simulink model "power_PSS"  (Simulink 6.0)
settings: Solver=ode23tb  StartTime=0.0  StopTime=20  MaxStep=1/60  RelTol=1e-4
undefined symbols (not defined in the file or in its folder): D1, Delta
libraries: powerlib x49, powerlib_extras x4
settings Model: Creator=rchampag  LastModifiedBy=batserve  ExtModeTrigMode=oneshot  ExtModeArmWhenConnect=off  ExtModeAutoUpdateStatusClock=off
settings DataIOCC: LimitDataPoints=off  SaveOutput=off  SaveTime=off  TimeSaveName=t  SignalLoggingName=sigsOut
settings OptimizationCC: BlockReduction=off  BooleanDataType=off
settings DebuggingCC: SolverPrmCheckMsg=none  UnconnectedOutputMsg=none
settings HardwareCC: TargetUnknown=on

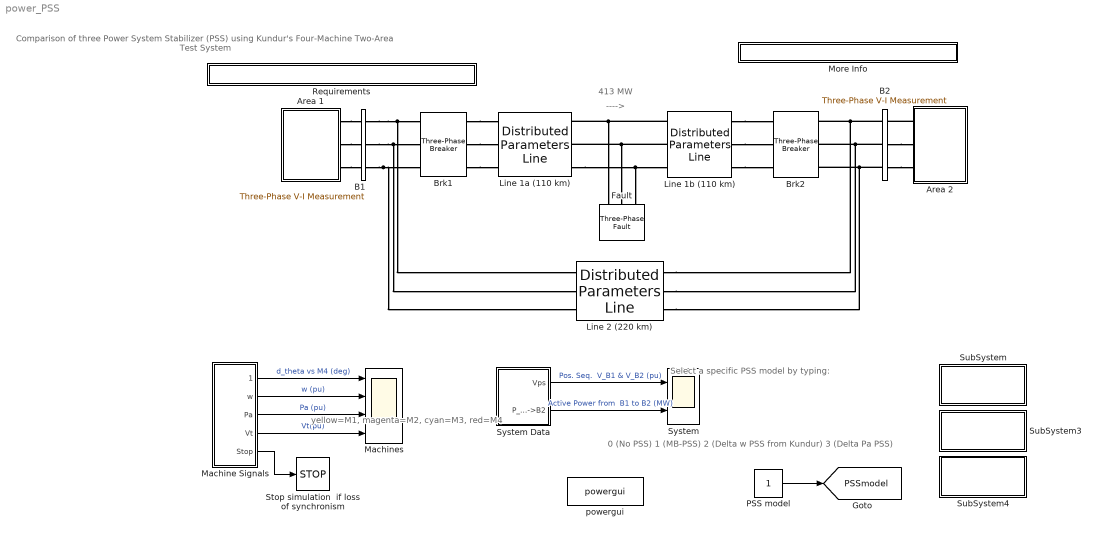
== system power_PSS ==
  note: Comparison of three Power System Stabilizer (PSS)
      | using Kundur's Four-Machine Two-Area Test System
  note: yellow=M1,
      | magenta=M2,
      | cyan=M3,
      | red=M4
  note: ---->
  note: 413 MW
  note: Select a specific PSS model
      | by typing:
  note: 0  (No PSS)
      | 1  (MB-PSS)
      | 2  (Delta w PSS from Kundur)
      | 3  (Delta Pa PSS)
  " Brk2" : powerlib/Elements/Three-Phase Breaker  InitialState=closed  SwitchA=on  SwitchB=on  SwitchC=on  SwitchTimes=[1+8/60]  External=off  BreakerResistance=0.001  SnubberResistance=1e6  SnubberCapacitance=0  Measurements=None
      settings: AttributesFormatString=\n
  Area 1 : Subsystem
  Area 2 : Subsystem
  B1 : powerlib/Measurements/Three-Phase V-I Measurement  VoltageMeasurement=phase-to-ground  SetLabelV=on  LabelV=Vabc_B1  Vpu=off  Vbase=500e3  CurrentMeasurement=yes  SetLabelI=on  LabelI=Iabc_B1  Ipu=off  Pbase=100e6  OutputType=Complex  PhasorSimulation=on  PSBequivalent=0
  B2 : powerlib/Measurements/Three-Phase V-I Measurement  VoltageMeasurement=phase-to-ground  SetLabelV=on  LabelV=Vabc_B2  Vpu=off  Vbase=500e3  CurrentMeasurement=yes  SetLabelI=on  LabelI=Iabc_B2  Ipu=off  Pbase=100e6  OutputType=Complex  PhasorSimulation=on  PSBequivalent=0
  Brk1 : powerlib/Elements/Three-Phase Breaker  InitialState=closed  SwitchA=on  SwitchB=on  SwitchC=on  SwitchTimes=[1+8/60]  External=off  BreakerResistance=0.001  SnubberResistance=inf  SnubberCapacitance=0  Measurements=None
      settings: AttributesFormatString=\n
  Fault : powerlib/Elements/Three-Phase Fault  Orientation=down  FaultA=on  FaultB=on  FaultC=on  FaultResistance=0.001  GroundFault=on  GroundResistance=0.001  External=off  SwitchStatus=[1 0]  SwitchTimes=[ 1 1+12/60]  InitialStates=[0 0 1]  SnubberResistance=inf  SnubberCapacitance=0  Measurements=None
  Line 1a (110 km) : powerlib/Elements/Distributed Parameters Line  Phases=3  Frequency=60  Resistance=[0.0001*529 1.61]  Inductance=[0.001*529/(377) 0.0061]  Capacitance=[0.00175/529/(377) 5.2489e-9]  Length=110  x1=[0 -1.08e-008 1.364e+005 -1.828e+005;0.0001245 -1.04e-008 1.448e+005 -1.762e+005;0.000249 -9.969e-009 1.529e+005 -1.692e+005;0.0003735 -9.519e-009 1.607e+005 -1.618e+005;0.0004979 -9.048e-009 1.681e+005 -1.541e+005;0.0006224 -8.557e-009 1.751e+005 -1.461e+005]  x2=[0 -8.707e-009 8.941e+004 -2.072e+005;0.0001245 -8.096e-009 9.903e+004 -2.027e+005;0.000249 -7.467e-009 1.084e+005 -1.979e+005;0.0003735 -6.821e-009 1.176e+005 -1.926e+005;0.0004979 -6.16e-009 1.265e+005 -1.868e+005;0.0006224 -5.486e-009 1.351e+005 -1.807e+005]  x3=[0 -1.712e-011 -188.2 278.4;0.0001245 -1.624e-011 -201 269.2;0.000249 -1.531e-011 -213.4 259.5;0.0003735 -1.435e-011 -225.4 249.2;0.0004979 -1.336e-011 -236.8 238.4;0.0006224 -1.234e-011 -247.8 227]  x4=[0 -1.348e-012 676.1 -1284;0.0001245 -1.525e-012 735.6 -1251;0.000249 -1.7e-012 793.5 -1215;0.0003735 -1.87e-012 849.6 -1176;0.0004979 -2.037e-012 903.8 -1135;0.0006224 -2.199e-012 956.1 -1091]  x5=0.0006224  Measurements=None
      settings: AttributesFormatString=\n
  Line 1b (110 km) : powerlib/Elements/Distributed Parameters Line  Phases=3  Frequency=60  Resistance=[0.0001*529 1.61]  Inductance=[0.001*529/(377) 0.0061]  Capacitance=[0.00175/529/(377) 5.2489e-9]  Length=110  x1=[0 -8.707e-009 8.941e+004 -2.072e+005;0.0001245 -8.096e-009 9.903e+004 -2.027e+005;0.000249 -7.467e-009 1.084e+005 -1.979e+005;0.0003735 -6.821e-009 1.176e+005 -1.926e+005;0.0004979 -6.16e-009 1.265e+005 -1.868e+005;0.0006224 -5.486e-009 1.351e+005 -1.807e+005]  x2=[0 -6.602e-009 4.098e+004 -2.27e+005;0.0001245 -5.796e-009 5.158e+004 -2.248e+005;0.000249 -4.976e-009 6.207e+004 -2.221e+005;0.0003735 -4.146e-009 7.242e+004 -2.19e+005;0.0004979 -3.306e-009 8.262e+004 -2.153e+005;0.0006224 -2.459e-009 9.263e+004 -2.112e+005]  x3=[0 -1.532e-011 -233.8 258.9;0.0001245 -1.425e-011 -245.7 247.7;0.000249 -1.315e-011 -257 235.9;0.0003735 -1.203e-011 -267.8 223.6;0.0004979 -1.088e-011 -278 210.7;0.0006224 -9.699e-012 -287.6 197.5]  x4=[0 -3.575e-013 477.8 -1356;0.0001245 -3.081e-013 540.9 -1332;0.000249 -2.58e-013 602.8 -1306;0.0003735 -2.073e-013 663.4 -1276;0.0004979 -1.562e-013 722.5 -1243;0.0006224 -1.047e-013 780 -1208]  x5=0.0006224  Measurements=None
      settings: AttributesFormatString=\n
  Line 2 (220 km) : powerlib/Elements/Distributed Parameters Line  Phases=3  Frequency=60  Resistance=[0.0001*529 1.61]  Inductance=[0.001*529/(377) 0.0061]  Capacitance=[0.00175/529/(377) 5.2489e-9]  Length=220  x1=[0 -1.135e-008 1.084e+005 -2.006e+005;0.000249 -1.036e-008 1.268e+005 -1.896e+005;0.0004979 -9.29e-009 1.44e+005 -1.769e+005;0.0007469 -8.134e-009 1.599e+005 -1.626e+005;0.0009959 -6.906e-009 1.745e+005 -1.469e+005;0.001245 -5.617e-009 1.875e+005 -1.299e+005]  x2=[0 -8.979e-009 7634 -2.305e+005;0.000249 -7.841e-009 2.92e+004 -2.288e+005;0.0004979 -6.634e-009 5.052e+004 -2.25e+005;0.0007469 -5.368e-009 7.139e+004 -2.193e+005;0.0009959 -4.055e-009 9.163e+004 -2.117e+005;0.001245 -2.707e-009 1.111e+005 -2.021e+005]  x3=[0 -1.027e-011 -145.5 302.4;0.000249 -9.359e-012 -173.2 287.5;0.0004979 -8.367e-012 -199.4 270;0.0007469 -7.303e-012 -223.8 250.1;0.0009959 -6.174e-012 -246.3 228;0.001245 -4.99e-012 -266.6 203.9]  x4=[0 -8.487e-012 273.7 -1399;0.000249 -8.24e-012 403.7 -1367;0.0004979 -7.92e-012 530 -1323;0.0007469 -7.531e-012 651.7 -1268;0.0009959 -7.075e-012 767.7 -1201;0.001245 -6.557e-012 876.9 -1124]  x5=0.001245  Measurements=None
      settings: AttributesFormatString=\n
  Machine Signals : Subsystem
  Machines : Scope  NumInputPorts=4
      settings: TimeRange=10  YMin=0~0.994~-0.35~0.95  YMax=130~1.005~0.2~1.175  SaveName=mach
  More Info : Subsystem
      settings: OpenFcn=web(which('psbpss.html'))
      mask Display: disp('? : Double click here for more info')
  PSS model : Constant
  Requirements : Subsystem  Description=|  LoadFcn=|  InitFcn=|
      LoadFcn=|
      | Toolboxes = ver;                                                                                                                 
      | installedtoolboxes = {Toolboxes.Name};                                                                                           
      | k = strcmp('Control System Toolbox',installedtoolboxes);                                                                         
      | if ~any(k)                                                                                                                       
      |     H = warndlg(['You need to install the Control System Toolbox in order to run the power_pss demo'],'SimPowerSystems warning');
      |     uiwait(H);                                                                                                                   
      | end
      InitFcn=|
      | Toolboxes = ver;                                                                                  
      | installedtoolboxes = {Toolboxes.Name};                                                            
      | k = strcmp('Control System Toolbox',installedtoolboxes);                                          
      | if ~any(k)                                                                                        
      |     error(['You need to install the Control System Toolbox in order to run the power_pss demo.']);
      | end
      Description=|
      | This block is used to popup errors and warnings if the
      | Control System Toolbox is not installed.
      settings: OpenFcn=|
      | Toolboxes = ver;
      | installedtoolboxes = {Toolboxes.Name};
      | k = strcmp('Control System Toolbox',installedtoolboxes);
      | if ~any(k)
      |     warndlg(['You need to install the Control System Toolbox in order to run the power_pss demo.'],'SimPowerSystems warning');
      |                                                                                                                                                         end
      mask Display: disp('This demo requires the Control System Toolbox')
  Stop simulation  if loss of synchronism : Stop
  SubSystem : Subsystem
      settings: OpenFcn=openfig('psbPSSbode.fig');
      mask Display: disp('Show Bode plot \nof PSS')
  SubSystem3 : Subsystem
      settings: OpenFcn=openfig('psbPSSstep.fig');
      mask Display: disp('Show results: \nStep on vref\nof M1')
  SubSystem4 : Subsystem
      settings: OpenFcn=openfig('psbPSSfault.fig');
      mask Display: disp('Show results: \n3-phase fault')
  System : Scope  NumInputPorts=2
      settings: TimeRange=10  YMin=0.9475~389  YMax=0.9675~401  SaveName=mach1
  System Data : Subsystem
  powergui : powerlib/powergui  Priority=2  Frange=logspace(0,3,50)  Ylog=off  Xlog=off  save=off  variable=ZData  ZoomFFT=on  StartTime=0.0  cycles=1  DisplayStyle=1  fundamental=60  FreqAxis=off  MaxFrequency=1000  frequencyindice=1  frequencyindicesteady=1  RmsSteady=1  display=off  Ts=0  methode=on  frequency=60  echomessages=on
  tag scope: PSSmodel=global
  wires:
  Machine Signals/1(d_theta) -> Machines/1  "d_theta vs M4 (deg)"
  Machine Signals/2(w) -> Machines/2  "w (pu)"
  Machine Signals/3(Pa) -> Machines/3  "Pa (pu)"
  Machine Signals/4(Vt) -> Machines/4  "Vt(pu)"
  Machine Signals/5(Stop) -> Stop simulation  if loss of synchronism/1
  System Data/1(Vps) -> System/1  "Pos. Seq.  V_B1 & V_B2 (pu)"
  System Data/2(P_B1->B2) -> System/2  "Active Power from  B1 to B2 (MW)"
  PSS model/1 -> [PSSmodel]
  connections:
  Brk1/RConn1 -- Line 1a (110 km)/LConn1
  Brk1/RConn2 -- Line 1a (110 km)/LConn2
  Brk1/RConn3 -- Line 1a (110 km)/LConn3
  Line 1b (110 km)/LConn1 -- Line 1a (110 km)/RConn1 -- Fault/LConn1
  Line 1b (110 km)/LConn2 -- Line 1a (110 km)/RConn2 -- Fault/LConn2
  Line 1a (110 km)/RConn3 -- Line 1b (110 km)/LConn3 -- Fault/LConn3
  Line 1b (110 km)/RConn1 -- " Brk2"/LConn1
  Line 1b (110 km)/RConn2 -- " Brk2"/LConn2
  Line 1b (110 km)/RConn3 -- " Brk2"/LConn3
  Area 1/RConn2 -- B1/LConn2
  Area 1/RConn1 -- B1/LConn1
  Area 1/RConn3 -- B1/LConn3
  B1/RConn2 -- Brk1/LConn2 -- Line 2 (220 km)/LConn2
  B1/RConn1 -- Brk1/LConn1 -- Line 2 (220 km)/LConn1
  B1/RConn3 -- Brk1/LConn3 -- Line 2 (220 km)/LConn3
  B2/RConn2 -- Area 2/LConn2
  Area 2/LConn1 -- B2/RConn1
  B2/RConn3 -- Area 2/LConn3
  B2/LConn2 -- " Brk2"/RConn2 -- Line 2 (220 km)/RConn2
  B2/LConn1 -- " Brk2"/RConn1 -- Line 2 (220 km)/RConn1
  B2/LConn3 -- " Brk2"/RConn3 -- Line 2 (220 km)/RConn3

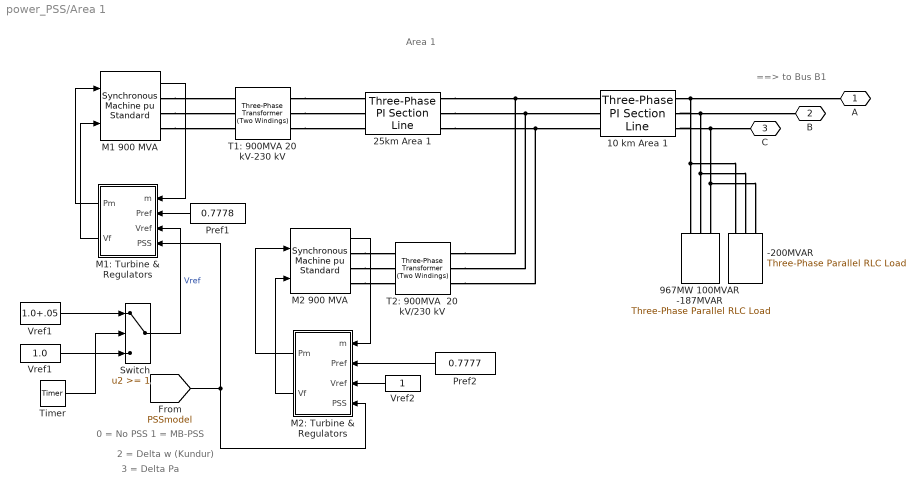
== system power_PSS/Area 1 ==
  note: Area 1
  note: ==> to Bus B1
  note: 0 = No PSS
      | 1 = MB-PSS
  note: 3 = Delta Pa
  note: 2 = Delta w (Kundur)
  -200MVAR : powerlib/Elements/Three-Phase Parallel RLC Load  Orientation=down  PhysicalDomain=powersysdomain  SubClassName=unknown  LeftPortType=p1  RightPortType=p1  LConnTagsString=A|B|C  Configuration=Y (grounded)  NominalVoltage=230e3  NominalFrequency=60  ActivePower=0  InductivePower=0  CapacitivePower=200e6  Measurements=None
  10 km Area 1 : powerlib/Elements/Three-Phase PI Section Line  PhysicalDomain=powersysdomain  SubClassName=unknown  LeftPortType=p1  RightPortType=p1  LConnTagsString=a|b|c  RConnTagsString=A|B|C  Frequency=60  Resistances=[0.0001*529 1.61]  Inductances=[0.001*529/(377) 0.0061]  Capacitances=[0.00175/529/(377) 5.2489e-9]  Length=10
  25km Area 1 : powerlib/Elements/Three-Phase PI Section Line  PhysicalDomain=powersysdomain  SubClassName=unknown  LeftPortType=p1  RightPortType=p1  LConnTagsString=a|b|c  RConnTagsString=A|B|C  Frequency=60  Resistances=[0.0001*529 1.61]  Inductances=[0.001*529/(377) 0.0061]  Capacitances=[0.00175/529/(377) 5.2489e-9]  Length=25
  967MW 100MVAR -187MVAR : powerlib/Elements/Three-Phase Parallel RLC Load  Orientation=down  PhysicalDomain=powersysdomain  SubClassName=unknown  LeftPortType=p1  RightPortType=p1  LConnTagsString=A|B|C  Configuration=Y (grounded)  NominalVoltage=230e3  NominalFrequency=60  ActivePower=967e6  InductivePower=100e6  CapacitivePower=187e6  Measurements=None
  M1 900 MVA : powerlib/Machines/Synchronous Machine pu Standard  PresetModel=No  ShowDetailedParameters=on  RotorType=Round  NominalParameters="[900E6  20000   60 ]"  Reactances1=[1.8 .3 .25 1.7 .55 .25 .2]  Reactances2=[ 1.305, 0.296, 0.252, 0.474, 0.243, 0.18 ]  dAxisTimeConstants=Open-circuit  qAxisTimeConstants=Open-circuit  TimeConstants1=[]  TimeConstants2=[8 .03 .4 .05]  TimeConstants3=[]  TimeConstants4=[]  TimeConstants5=[ 1.01, 0.053, 0.1 ]  TimeConstants6=[]  TimeConstants7=[]  TimeConstants8=[]  StatorResistance=0.0025  Mechanical="[ 6.5 0  4]"  InitialConditions=[0 -31.4247 0.784453 0.784453 0.784453 2.7401 -117.26 122.74 1.83395]  SetSaturation=off  Saturation=[0.6404,0.7127,0.8441,0.9214,0.9956,1.082,1.19,1.316,1.457;0.7,0.7698,0.8872,0.9466,0.9969,1.046,1.1,1.151,1.201]  Units=0.5  LoadFlowParameters=[1 700000000 0 0 0]
      settings: AttributesFormatString=\n\n
  M1: Turbine & Regulators : Subsystem  Orientation=left
  M2 900 MVA : powerlib/Machines/Synchronous Machine pu Standard  PresetModel=No  ShowDetailedParameters=on  RotorType=Round  NominalParameters="[900E6  20000   60 ]"  Reactances1=[1.8 .3 .25 1.7 .55 .25 .2]  Reactances2=[ 1.305, 0.296, 0.252, 0.474, 0.243, 0.18 ]  dAxisTimeConstants=Open-circuit  qAxisTimeConstants=Open-circuit  TimeConstants1=[]  TimeConstants2=[8 .03 .4 .05]  TimeConstants3=[]  TimeConstants4=[]  TimeConstants5=[ 1.01, 0.053, 0.1 ]  TimeConstants6=[]  TimeConstants7=[]  TimeConstants8=[]  StatorResistance=0.0025  Mechanical="[ 6.5 0  4]"  InitialConditions=[0 -42.8075 0.788608 0.788608 0.788608 -9.54571 -129.546 110.454 1.86756]  SetSaturation=off  Saturation=[0.6404,0.7127,0.8441,0.9214,0.9956,1.082,1.19,1.316,1.457;0.7,0.7698,0.8872,0.9466,0.9969,1.046,1.1,1.151,1.201]  Units=0.5  LoadFlowParameters=[2 700000000 0 0 0]
      settings: AttributesFormatString=\n\n
  M2: Turbine & Regulators : Subsystem  Orientation=left
  Pref1 : Constant  Orientation=left  Value=0.7778
  Pref2 : Constant  Orientation=left  Value=0.7777
  Switch : Switch  Threshold=1  InputSameDT=on
  T1: 900MVA 20 kV-230 kV : powerlib/Elements/Three-Phase Transformer (Two Windings)  NominalPower="[ 900e6   60 ]"  Winding1Connection=Delta (D1)  Winding1="[ 20e3  1e-6   0  ]"  Winding2Connection=Yg  Winding2="[ 230e3  1e-6   0.15 ]"  SetSaturation=off  Rm=500  Lm=500  Saturation="[ 0,0  ;  0.005,1.2  ;  1.0,1.4 ]"  Hysteresis=off  DataFile='hysteresis'  SetInitialFlux=off  InitialFluxes=[ 0.8 , -0.8 , 0.7 ]  Measurements=None  TransfoNumber=0
  T2: 900MVA  20 kV/230 kV : powerlib/Elements/Three-Phase Transformer (Two Windings)  NominalPower=[ 900e6 60 ]  Winding1Connection=Delta (D1)  Winding1="[ 20e3 1e-6  0.0]"  Winding2Connection=Yg  Winding2=[ 230e3 1e-6 0.15]  SetSaturation=off  Rm=500  Lm=500  Saturation="[ 0,0  ;  0.005,1.2  ;  1.0,1.4 ]"  Hysteresis=off  DataFile='hysteresis'  SetInitialFlux=off  InitialFluxes=[ 0.8 , -0.8 , 0.7 ]  Measurements=None  TransfoNumber=0
  Timer : powerlib_extras/Control  Blocks/Timer  t=[0 1 1.2]*100  e=[0 1 0 ]
  Vref1 : Constant  Value=1.0
  "Vref1 " : Constant  Value=1.0+.05
  Vref2 : Constant  Orientation=left
  " A" : PMIOPort  Orientation=left  Port=1  Side=Right
  " B" : PMIOPort  Orientation=left  Port=2  Side=Right
  " C" : PMIOPort  Orientation=left  Port=3  Side=Right
  wires:
  Pref1/1 -> M1: Turbine & Regulators/2(Pref)
  Switch/1 -> M1: Turbine & Regulators/3(Vref)  "Vref"
  Timer/1 -> Switch/2
  [PSSmodel] -> M1: Turbine & Regulators/4(PSS), M2: Turbine & Regulators/4(PSS)
  Pref2/1 -> M2: Turbine & Regulators/2(Pref)
  Vref2/1 -> M2: Turbine & Regulators/3(Vref)
  Vref1/1 -> Switch/3
  "Vref1 "/1 -> Switch/1
  M2 900 MVA/1 -> M2: Turbine & Regulators/1(m)
  M2: Turbine & Regulators/1(Pm) -> M2 900 MVA/1
  M2: Turbine & Regulators/2(Vf) -> M2 900 MVA/2
  M1: Turbine & Regulators/1(Pm) -> M1 900 MVA/1
  M1: Turbine & Regulators/2(Vf) -> M1 900 MVA/2
  M1 900 MVA/1 -> M1: Turbine & Regulators/1(m)
  connections:
  T1: 900MVA 20 kV-230 kV/RConn1 -- 25km Area 1/LConn1
  T1: 900MVA 20 kV-230 kV/RConn2 -- 25km Area 1/LConn2
  M2 900 MVA/RConn1 -- T2: 900MVA  20 kV/230 kV/LConn1
  M2 900 MVA/RConn2 -- T2: 900MVA  20 kV/230 kV/LConn2
  M2 900 MVA/RConn3 -- T2: 900MVA  20 kV/230 kV/LConn3
  T1: 900MVA 20 kV-230 kV/RConn3 -- 25km Area 1/LConn3
  10 km Area 1/RConn1 -- " A"/RConn1 -- 967MW 100MVAR -187MVAR/LConn1 -- -200MVAR/LConn1
  10 km Area 1/RConn2 -- " B"/RConn1 -- 967MW 100MVAR -187MVAR/LConn2 -- -200MVAR/LConn2
  10 km Area 1/RConn3 -- " C"/RConn1 -- 967MW 100MVAR -187MVAR/LConn3 -- -200MVAR/LConn3
  M1 900 MVA/RConn1 -- T1: 900MVA 20 kV-230 kV/LConn1
  M1 900 MVA/RConn2 -- T1: 900MVA 20 kV-230 kV/LConn2
  M1 900 MVA/RConn3 -- T1: 900MVA 20 kV-230 kV/LConn3
  25km Area 1/RConn2 -- 10 km Area 1/LConn2 -- T2: 900MVA  20 kV/230 kV/RConn2
  25km Area 1/RConn1 -- 10 km Area 1/LConn1 -- T2: 900MVA  20 kV/230 kV/RConn1
  25km Area 1/RConn3 -- 10 km Area 1/LConn3 -- T2: 900MVA  20 kV/230 kV/RConn3

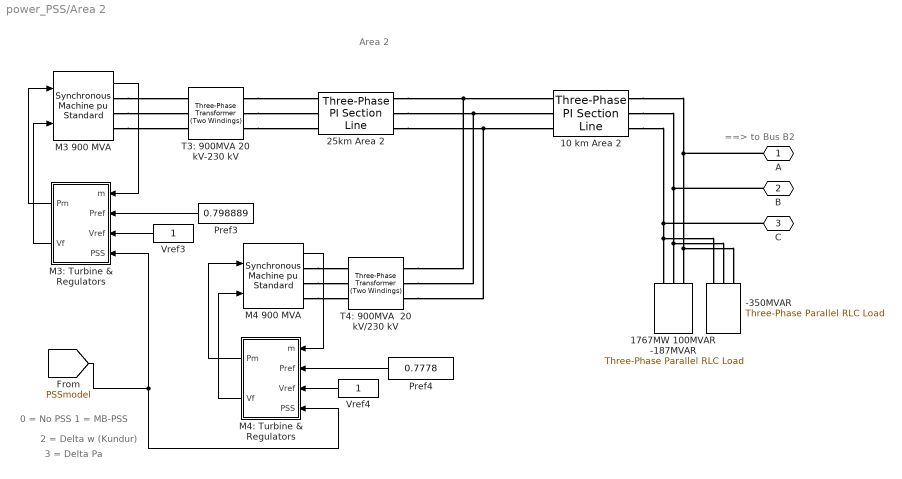
== system power_PSS/Area 2 ==
  note: 2 = Delta w (Kundur)
  note: 3 = Delta Pa
  note: 0 = No PSS
      | 1 = MB-PSS
  note: ==> to Bus B2
  note: Area 2
  -350MVAR : powerlib/Elements/Three-Phase Parallel RLC Load  Orientation=down  PhysicalDomain=powersysdomain  SubClassName=unknown  LeftPortType=p1  RightPortType=p1  LConnTagsString=A|B|C  Configuration=Y (grounded)  NominalVoltage=230e3  NominalFrequency=60  ActivePower=0  InductivePower=0  CapacitivePower=350e6  Measurements=None
  10 km Area 2 : powerlib/Elements/Three-Phase PI Section Line  PhysicalDomain=powersysdomain  SubClassName=unknown  LeftPortType=p1  RightPortType=p1  LConnTagsString=a|b|c  RConnTagsString=A|B|C  Frequency=60  Resistances=[0.0001*529 1.61]  Inductances=[0.001*529/(377) 0.0061]  Capacitances=[0.00175/529/(377) 5.2489e-9]  Length=10
  1767MW 100MVAR -187MVAR : powerlib/Elements/Three-Phase Parallel RLC Load  Orientation=down  PhysicalDomain=powersysdomain  SubClassName=unknown  LeftPortType=p1  RightPortType=p1  LConnTagsString=A|B|C  Configuration=Y (grounded)  NominalVoltage=230e3  NominalFrequency=60  ActivePower=1767e6  InductivePower=100e6  CapacitivePower=187e6  Measurements=None
  25km Area 2 : powerlib/Elements/Three-Phase PI Section Line  PhysicalDomain=powersysdomain  SubClassName=unknown  LeftPortType=p1  RightPortType=p1  LConnTagsString=a|b|c  RConnTagsString=A|B|C  Frequency=60  Resistances=[0.0001*529 1.61]  Inductances=[0.001*529/(377) 0.0061]  Capacitances=[0.00175/529/(377) 5.2489e-9]  Length=25
  M3 900 MVA : powerlib/Machines/Synchronous Machine pu Standard  PresetModel=No  ShowDetailedParameters=on  RotorType=Round  NominalParameters="[900E6  20000   60 ]"  Reactances1=[1.8 .3 .25 1.7 .55 .25 .2]  Reactances2=[ 1.305, 0.296, 0.252, 0.474, 0.243, 0.18 ]  dAxisTimeConstants=Open-circuit  qAxisTimeConstants=Open-circuit  TimeConstants1=[]  TimeConstants2=[8 .03 .4 .05]  TimeConstants3=[]  TimeConstants4=[]  TimeConstants5=[ 1.01, 0.053, 0.1 ]  TimeConstants6=[]  TimeConstants7=[]  TimeConstants8=[]  StatorResistance=0.0025  Mechanical="[ 6.175 0  4]"  InitialConditions=[0 -56.3243 0.8041 0.8041 0.8041 -22.4087 -142.409 97.5913 1.85092]  SetSaturation=off  Saturation=[0.6404,0.7127,0.8441,0.9214,0.9956,1.082,1.19,1.316,1.457;0.7,0.7698,0.8872,0.9466,0.9969,1.046,1.1,1.151,1.201]  Units=0.5  LoadFlowParameters=[1 719000000 0 0 0]
      settings: AttributesFormatString=\n\n
  M3: Turbine & Regulators : Subsystem  Orientation=left
  M4 900 MVA : powerlib/Machines/Synchronous Machine pu Standard  PresetModel=No  ShowDetailedParameters=on  RotorType=Round  NominalParameters="[900E6  20000   60 ]"  Reactances1=[1.8 .3 .25 1.7 .55 .25 .2]  Reactances2=[ 1.305, 0.296, 0.252, 0.474, 0.243, 0.18 ]  dAxisTimeConstants=Open-circuit  qAxisTimeConstants=Open-circuit  TimeConstants1=[]  TimeConstants2=[8 .03 .4 .05]  TimeConstants3=[]  TimeConstants4=[]  TimeConstants5=[ 1.01, 0.053, 0.1 ]  TimeConstants6=[]  TimeConstants7=[]  TimeConstants8=[]  StatorResistance=0.0025  Mechanical="[ 6.175 0  4]"  InitialConditions=[0 -67.7513 0.783185 0.783185 0.783185 -33.268 -153.268 86.732 1.82209]  SetSaturation=off  Saturation=[0.6404,0.7127,0.8441,0.9214,0.9956,1.082,1.19,1.316,1.457;0.7,0.7698,0.8872,0.9466,0.9969,1.046,1.1,1.151,1.201]  Units=0.5  LoadFlowParameters=[1 700000000 0 0 0]
      settings: AttributesFormatString=\n\n
  M4: Turbine & Regulators : Subsystem  Orientation=left
  Pref3 : Constant  Orientation=left  Value=0.798889
  Pref4 : Constant  Orientation=left  Value=0.7778
  T3: 900MVA 20 kV-230 kV : powerlib/Elements/Three-Phase Transformer (Two Windings)  NominalPower="[ 900e6   60 ]"  Winding1Connection=Delta (D1)  Winding1="[ 20e3  1e-6   0  ]"  Winding2Connection=Yg  Winding2="[ 230e3  1e-6   0.15 ]"  SetSaturation=off  Rm=500  Lm=500  Saturation="[ 0,0  ;  0.005,1.2  ;  1.0,1.4 ]"  Hysteresis=off  DataFile='hysteresis'  SetInitialFlux=off  InitialFluxes=[ 0.8 , -0.8 , 0.7 ]  Measurements=None  TransfoNumber=0
  T4: 900MVA  20 kV/230 kV : powerlib/Elements/Three-Phase Transformer (Two Windings)  NominalPower=[ 900e6 60 ]  Winding1Connection=Delta (D1)  Winding1="[ 20e3 1e-6  0.0]"  Winding2Connection=Yg  Winding2=[ 230e3 1e-6 0.15]  SetSaturation=off  Rm=500  Lm=500  Saturation="[ 0,0  ;  0.005,1.2  ;  1.0,1.4 ]"  Hysteresis=off  DataFile='hysteresis'  SetInitialFlux=off  InitialFluxes=[ 0.8 , -0.8 , 0.7 ]  Measurements=None  TransfoNumber=0
  Vref3 : Constant  Orientation=left
  Vref4 : Constant  Orientation=left
  A : PMIOPort  Orientation=left  Port=1  Side=Left
  B : PMIOPort  Orientation=left  Port=2  Side=Left
  C : PMIOPort  Orientation=left  Port=3  Side=Left
  wires:
  [PSSmodel] -> M3: Turbine & Regulators/4(PSS), M4: Turbine & Regulators/4(PSS)
  Pref3/1 -> M3: Turbine & Regulators/2(Pref)
  Vref3/1 -> M3: Turbine & Regulators/3(Vref)
  Pref4/1 -> M4: Turbine & Regulators/2(Pref)
  Vref4/1 -> M4: Turbine & Regulators/3(Vref)
  M3 900 MVA/1 -> M3: Turbine & Regulators/1(m)
  M3: Turbine & Regulators/2(Vf) -> M3 900 MVA/2
  M3: Turbine & Regulators/1(Pm) -> M3 900 MVA/1
  M4: Turbine & Regulators/1(Pm) -> M4 900 MVA/1
  M4: Turbine & Regulators/2(Vf) -> M4 900 MVA/2
  M4 900 MVA/1 -> M4: Turbine & Regulators/1(m)
  connections:
  M3 900 MVA/RConn3 -- T3: 900MVA 20 kV-230 kV/LConn3
  M3 900 MVA/RConn2 -- T3: 900MVA 20 kV-230 kV/LConn2
  M3 900 MVA/RConn1 -- T3: 900MVA 20 kV-230 kV/LConn1
  T3: 900MVA 20 kV-230 kV/RConn3 -- 25km Area 2/LConn3
  M4 900 MVA/RConn3 -- T4: 900MVA  20 kV/230 kV/LConn3
  M4 900 MVA/RConn2 -- T4: 900MVA  20 kV/230 kV/LConn2
  M4 900 MVA/RConn1 -- T4: 900MVA  20 kV/230 kV/LConn1
  T3: 900MVA 20 kV-230 kV/RConn2 -- 25km Area 2/LConn2
  T3: 900MVA 20 kV-230 kV/RConn1 -- 25km Area 2/LConn1
  10 km Area 2/RConn1 -- A/RConn1 -- 1767MW 100MVAR -187MVAR/LConn3 -- -350MVAR/LConn3
  10 km Area 2/RConn2 -- B/RConn1 -- 1767MW 100MVAR -187MVAR/LConn2 -- -350MVAR/LConn2
  10 km Area 2/RConn3 -- C/RConn1 -- 1767MW 100MVAR -187MVAR/LConn1 -- -350MVAR/LConn1
  25km Area 2/RConn2 -- 10 km Area 2/LConn2 -- T4: 900MVA  20 kV/230 kV/RConn2
  25km Area 2/RConn1 -- 10 km Area 2/LConn1 -- T4: 900MVA  20 kV/230 kV/RConn1
  25km Area 2/RConn3 -- 10 km Area 2/LConn3 -- T4: 900MVA  20 kV/230 kV/RConn3

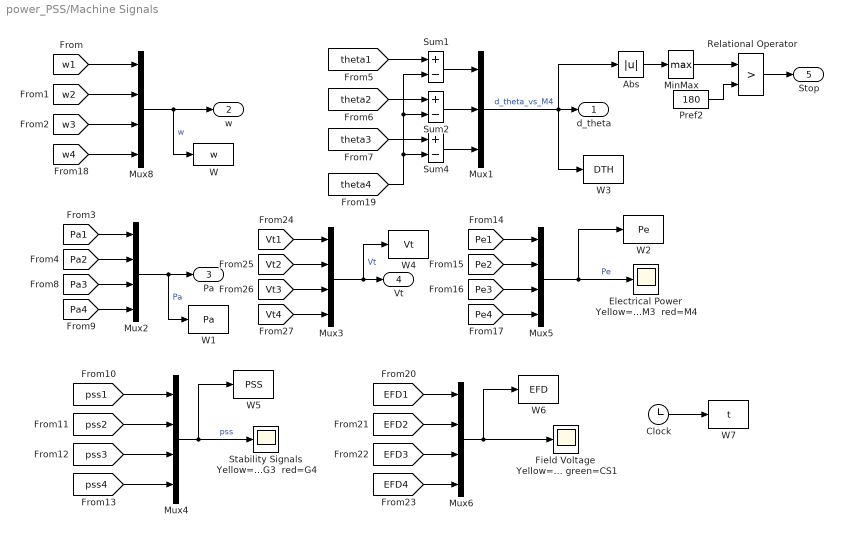
== system power_PSS/Machine Signals ==
  Abs : Abs  SaturateOnIntegerOverflow=on
  Clock : Clock
      settings: Decimation=10
  "Electrical Power  Yellow=M1 mag=M2 cyan=M3  red=M4 " : Scope
      settings: YMin=0.3  YMax=1
  Field Voltage  Yellow=G1 mag=G2 cyan=G3  red=G4 green=CS1 : Scope
      settings: YMin=1.845  YMax=1.96  SaveName=ScopeData4
  MinMax : MinMax  Function=max  SaturateOnIntegerOverflow=on  InputSameDT=on
  Mux1 : Mux  Inputs=3
  Mux{2..6,8} (6 alike) : Mux
  Pref2 : Constant  Value=180
  Relational Operator : RelationalOperator  Operator=>  InputSameDT=on
  "Stability Signals  Yellow=G1 mag=G2 cyan=G3  red=G4 " : Scope
      settings: YMin=-0.15  YMax=0.15  SaveName=ScopeData3
  Sum1 : Sum  Inputs=+-  SaturateOnIntegerOverflow=on  InputSameDT=on
  Sum2 : Sum  Inputs=+-  SaturateOnIntegerOverflow=on  InputSameDT=on
  Sum4 : Sum  Inputs=+-  SaturateOnIntegerOverflow=on  InputSameDT=on
  W : ToWorkspace  VariableName=w  SampleTime=1/60  SaveFormat=Array
  W1 : ToWorkspace  VariableName=Pa  SampleTime=1/60  SaveFormat=Array
  W2 : ToWorkspace  VariableName=Pe  SampleTime=1/60  SaveFormat=Array
  W3 : ToWorkspace  VariableName=DTH  SampleTime=1/60  SaveFormat=Array
  W4 : ToWorkspace  VariableName=Vt  SampleTime=1/60  SaveFormat=Array
  W5 : ToWorkspace  VariableName=PSS  SampleTime=1/60  SaveFormat=Array
  W6 : ToWorkspace  VariableName=EFD  SampleTime=1/60  SaveFormat=Array
  W7 : ToWorkspace  VariableName=t  SampleTime=1/60  SaveFormat=Array
  d_theta : Outport
  w : Outport  Port=2
  Pa : Outport  Port=3
  Vt : Outport  Port=4
  Stop : Outport  Port=5
  wires:
  Mux1/1 -> d_theta/1, Abs/1, W3/1  "d_theta_vs_M4"
  Abs/1 -> MinMax/1
  Pref2/1 -> Relational Operator/2
  MinMax/1 -> Relational Operator/1
  [Pa1] -> Mux2/1
  Mux4/1 -> "Stability Signals  Yellow=G1 mag=G2 cyan=G3  red=G4 "/1, W5/1  "pss"
  [pss1] -> Mux4/1
  [pss2] -> Mux4/2
  [pss4] -> Mux4/4
  [pss3] -> Mux4/3
  [EFD1] -> Mux6/1
  [EFD2] -> Mux6/2
  [EFD4] -> Mux6/4
  [EFD3] -> Mux6/3
  Mux6/1 -> Field Voltage  Yellow=G1 mag=G2 cyan=G3  red=G4 green=CS1/1, W6/1
  Mux8/1 -> w/1, W/1  "w"
  Relational Operator/1 -> Stop/1
  Mux2/1 -> Pa/1, W1/1  "Pa"
  [theta1] -> Sum1/1
  Sum1/1 -> Mux1/1
  [theta2] -> Sum2/1
  [theta3] -> Sum4/1
  [theta4] -> Sum4/2, Sum2/2, Sum1/2
  Sum2/1 -> Mux1/2
  Sum4/1 -> Mux1/3
  [Pa2] -> Mux2/2
  [Pa3] -> Mux2/3
  [Pa4] -> Mux2/4
  [Vt1] -> Mux3/1
  [Vt2] -> Mux3/2
  [Vt3] -> Mux3/3
  [Vt4] -> Mux3/4
  Mux3/1 -> Vt/1, W4/1  "Vt"
  [Pe1] -> Mux5/1
  [Pe2] -> Mux5/2
  [Pe3] -> Mux5/3
  [Pe4] -> Mux5/4
  Mux5/1 -> "Electrical Power  Yellow=M1 mag=M2 cyan=M3  red=M4 "/1, W2/1  "Pe"
  [w1] -> Mux8/1
  [w2] -> Mux8/2
  [w3] -> Mux8/3
  [w4] -> Mux8/4
  Clock/1 -> W7/1

== system power_PSS/More Info ==

== system power_PSS/Requirements ==

== system power_PSS/SubSystem ==

== system power_PSS/SubSystem3 ==

== system power_PSS/SubSystem4 ==

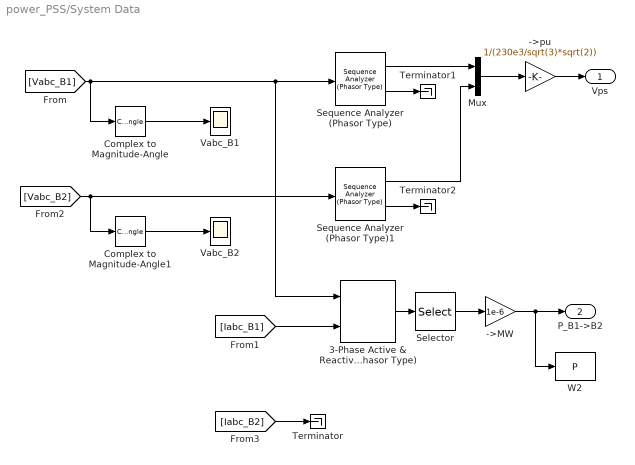
== system power_PSS/System Data ==
  ->MW : Gain  Gain=1e-6  SaturateOnIntegerOverflow=on
  ->pu : Gain  Gain=1/(230e3/sqrt(3)*sqrt(2))  SaturateOnIntegerOverflow=on
  3-Phase Active & Reactive Power (Phasor Type) : powerlib_extras/Phasor Library/3-Phase Active & Reactive Power (Phasor Type)
  Complex to Magnitude-Angle : ComplexToMagnitudeAngle  Output=Magnitude
  Complex to Magnitude-Angle1 : ComplexToMagnitudeAngle  Output=Magnitude
  Mux : Mux  Inputs=2
  Selector : Selector  InputPortWidth=2
  Sequence Analyzer (Phasor Type) : powerlib_extras/Phasor Library/Sequence Analyzer (Phasor Type)  seq=Positive
  Sequence Analyzer (Phasor Type)1 : powerlib_extras/Phasor Library/Sequence Analyzer (Phasor Type)  seq=Positive
  Terminator : Terminator
  Terminator1 : Terminator
  Terminator2 : Terminator
  Vabc_B1 : Scope
      settings: TimeRange=10  YMin=20  YMax=90  SaveName=mach2
  Vabc_B2 : Scope
      settings: TimeRange=10  YMin=20  YMax=90  SaveName=mach3
  W2 : ToWorkspace  VariableName=P  SampleTime=1/60  SaveFormat=Array
  Vps : Outport
  P_B1->B2 : Outport  Port=2
  wires:
  [Vabc_B1] -> Sequence Analyzer (Phasor Type)/1, 3-Phase Active & Reactive Power (Phasor Type)/1, Complex to Magnitude-Angle/1
  [Vabc_B2] -> Sequence Analyzer (Phasor Type)1/1, Complex to Magnitude-Angle1/1
  [Iabc_B2] -> Terminator/1
  Sequence Analyzer (Phasor Type)/2 -> Terminator1/1
  Sequence Analyzer (Phasor Type)1/2 -> Terminator2/1
  Sequence Analyzer (Phasor Type)1/1 -> Mux/2
  [Iabc_B1] -> 3-Phase Active & Reactive Power (Phasor Type)/2
  3-Phase Active & Reactive Power (Phasor Type)/1 -> Selector/1
  ->pu/1 -> Vps/1
  Sequence Analyzer (Phasor Type)/1 -> Mux/1
  Mux/1 -> ->pu/1
  ->MW/1 -> P_B1->B2/1, W2/1
  Complex to Magnitude-Angle/1 -> Vabc_B1/1
  Complex to Magnitude-Angle1/1 -> Vabc_B2/1
  Selector/1 -> ->MW/1

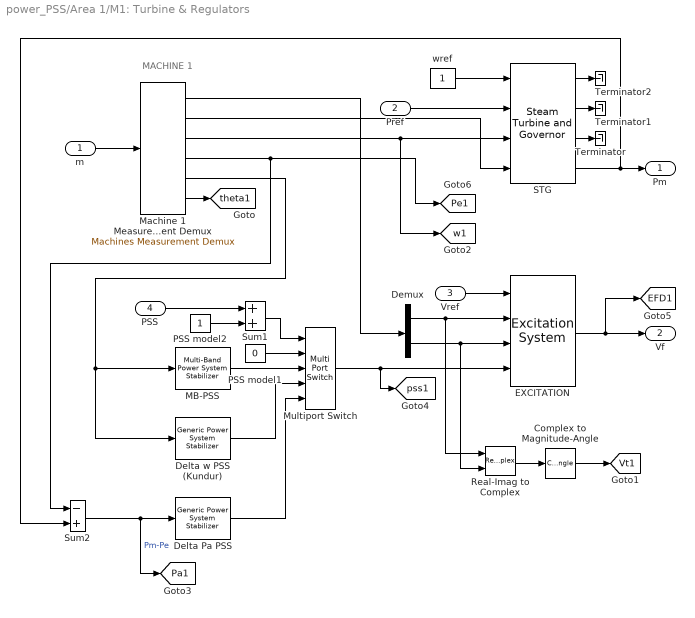
== system power_PSS/Area 1/M1: Turbine & Regulators ==
  note: MACHINE 1
  m : Inport  Port=1  LatchInput=off
  Pref : Inport  Port=2  LatchInput=off
  Vref : Inport  Port=3  LatchInput=off
  PSS : Inport  Port=4  LatchInput=off
  Complex to Magnitude-Angle : ComplexToMagnitudeAngle  Output=Magnitude
  "Delta Pa PSS " : powerlib/Machines/Generic Power System Stabilizer  Tsensor=15e-3  K=2.5*1.25  Twashout=1  Tleadlag1=[60e-3 1]  Tleadlag2=[0 0]  VSlimits=[-0.15 0.15]  Vinit=0  Plot_On=off  MagdB_On=off  FreqRange=logspace(-2,2,500)
  "Delta w PSS (Kundur) " : powerlib/Machines/Generic Power System Stabilizer  Tsensor=15e-3  K=30  Twashout=10  Tleadlag1=[50e-3 20e-3]  Tleadlag2=[3 5.4]  VSlimits=[-0.15 0.15]  Vinit=0  Plot_On=off  MagdB_On=off  FreqRange=logspace(-2,2,500)
  Demux : Demux  Outputs=2
  EXCITATION : powerlib/Machines/Excitation System  tr=20e-3  reg=[ 200, 0.001 ]  exc=[ 1, 0 ]  tgr=[ 0, 0 ]  damp=[ 0, 0 ]  sat=[ 0, 0 ]  lim=[ 0 , 12.3, 0 ]  v0=[1,1.83395]
  "MB-PSS " : powerlib/Machines/Multi-Band Power System Stabilizer  OperationMode=Simplified settings  Kg=1.0  GL=[0.2 30]  GI=[1.25 40]  GH=[12.0 160]  GLd=[66 66 9.4]  TcLF=[1.667 2 0 0 0 0 2 2.4 0 0 0 0 1 1]  GId=[66 66 47.6]  TcIF=[1 1 0.25 0.3 0 0 1 1 0.3 0.36 0 0 0 0]  GHd=[66 66 233]  TcHF="[0.01 0.012 0 0 0 0  0.012 0.0144 0 0 0 0 1 1]"  LIM=[.075 .15 .15 .15]  Plot_On=off  MagdB_On=off  FreqRange=logspace(-2,2,500)
  Machine 1 Measurement Demux : powerlib/Machines/Machines Measurement Demux  machType=Synchronous  ssm1=on  ssm2=on  ssm3=on  ssm4=on  ssm5=on  ssm6=on  sm1=off  sm2=off  sm3=off  sm4=off  sm5=off  sm6=on  sm7=on  sm8=on  sm9=on  sm10=on  sm11=on  sm115=off  sm12=off  sm13=off  sm14=off  asm1=on  asm2=on  asm3=on  asm4=on  asm5=on  asm6=on  asm7=on  asm8=on  asm9=on  asm10=on  asm11=on  pmsm1=on  pmsm2=on  pmsm3=on  pmsm4=on  pmsm5=on  pmsm6=on  lastType=2
  Multiport Switch : MultiPortSwitch  InputSameDT=on
  PSS model1 : Constant  Value=0
  PSS model2 : Constant
  Real-Imag to Complex : RealImagToComplex
  STG : powerlib/Machines/Steam Turbine and Governor  gentype=Tandem-compound (single mass)  reg1="[ 1  0.05    0 ]"  reg2="[ 0.001  0.15 ]"  reg3="[ -0.1  0.1  0  4.496 ]"  turb1="[ 0  10   3.3   0.5   ]"  turb2="[   0   0.36    0.36   0.28   ]"  HA="[ 0.046  1.430  1.465   0.192 ]"  KA="[ 90.44  53.88  64.59   62.94  ]"  DA="[ 0.0115  0.3575  0.3663   0.0137  ]"  ini1=0.7778  ini2=[0.779316,-31.4247]
  Sum1 : Sum  SaturateOnIntegerOverflow=on  InputSameDT=on
  Sum2 : Sum  Inputs=-+  SaturateOnIntegerOverflow=on  InputSameDT=on
  Terminator : Terminator
  Terminator1 : Terminator
  Terminator2 : Terminator
  wref : Constant
  Pm : Outport  InitialOutput=0
  Vf : Outport  Port=2  InitialOutput=0
  tag scope: EFD1=global, Pa1=global, Pe1=global, Vt1=global, pss1=global, theta1=global, w1=global
  wires:
  Demux/1 -> Real-Imag to Complex/1, EXCITATION/2
  Demux/2 -> Real-Imag to Complex/2, EXCITATION/3
  wref/1 -> STG/1
  Pref/1 -> STG/2
  m/1 -> Machine 1 Measurement Demux/1
  Vref/1 -> EXCITATION/1
  Real-Imag to Complex/1 -> Complex to Magnitude-Angle/1
  EXCITATION/1 -> Vf/1, [EFD1]
  Complex to Magnitude-Angle/1 -> [Vt1]
  Machine 1 Measurement Demux/6 -> [theta1]
  Multiport Switch/1 -> EXCITATION/4, [pss1]
  PSS model1/1 -> Multiport Switch/2
  "MB-PSS "/1 -> Multiport Switch/3
  "Delta w PSS (Kundur) "/1 -> Multiport Switch/4
  "Delta Pa PSS "/1 -> Multiport Switch/5
  PSS model2/1 -> Sum1/2
  Sum1/1 -> Multiport Switch/1
  PSS/1 -> Sum1/1
  Machine 1 Measurement Demux/1 -> Demux/1
  Machine 1 Measurement Demux/3 -> [w1], STG/3
  Machine 1 Measurement Demux/4 -> Sum2/1, [Pe1]
  Machine 1 Measurement Demux/5 -> "Delta w PSS (Kundur) "/1, "MB-PSS "/1
  Sum2/1 -> [Pa1], "Delta Pa PSS "/1  "Pm-Pe"
  STG/3 -> Terminator/1
  Machine 1 Measurement Demux/2 -> STG/4
  STG/4 -> Pm/1, Sum2/2
  STG/2 -> Terminator1/1
  STG/1 -> Terminator2/1

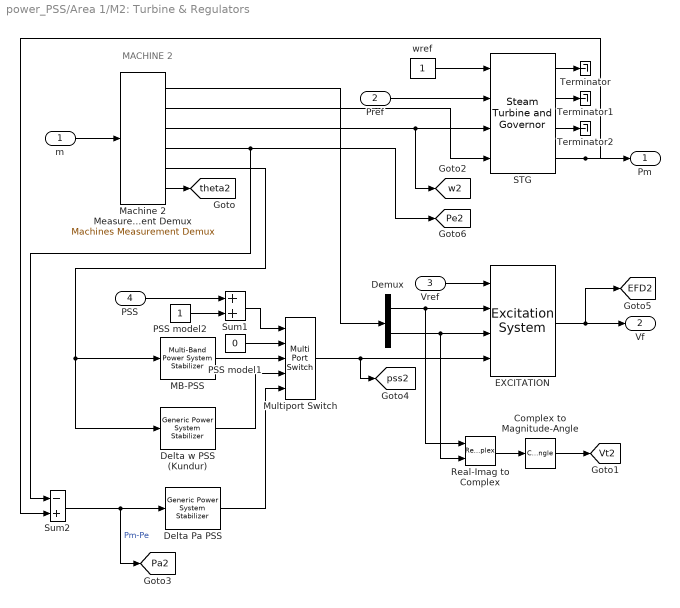
== system power_PSS/Area 1/M2: Turbine & Regulators ==
  note: MACHINE 2
  m : Inport  Port=1  LatchInput=off
  Pref : Inport  Port=2  LatchInput=off
  Vref : Inport  Port=3  LatchInput=off
  PSS : Inport  Port=4  LatchInput=off
  Complex to Magnitude-Angle : ComplexToMagnitudeAngle  Output=Magnitude
  "Delta Pa PSS " : powerlib/Machines/Generic Power System Stabilizer  Tsensor=15e-3  K=2.5*1.25  Twashout=1  Tleadlag1=[60e-3 1]  Tleadlag2=[0 0]  VSlimits=[-0.15 0.15]  Vinit=0  Plot_On=off  MagdB_On=on  FreqRange=logspace(-2,2,500)
  "Delta w PSS (Kundur) " : powerlib/Machines/Generic Power System Stabilizer  Tsensor=15e-3  K=30  Twashout=10  Tleadlag1=[50e-3 20e-3]  Tleadlag2=[3 5.4]  VSlimits=[-0.15 0.15]  Vinit=0  Plot_On=off  MagdB_On=on  FreqRange=logspace(-2,2,500)
  Demux : Demux  Outputs=2
  EXCITATION : powerlib/Machines/Excitation System  tr=20e-3  reg=[ 200, 0.001 ]  exc=[ 1, 0 ]  tgr=[ 0, 0 ]  damp=[ 0, 0 ]  sat=[ 0, 0 ]  lim=[ 0 , 12.3, 0 ]  v0=[1,1.86756]
  "MB-PSS " : powerlib/Machines/Multi-Band Power System Stabilizer  OperationMode=Simplified settings  Kg=1.0  GL=[0.2 30]  GI=[1.25 40]  GH=[12.0 160]  GLd=[66 66 9.4]  TcLF=[1.667 2 0 0 0 0 2 2.4 0 0 0 0 1 1]  GId=[66 66 47.6]  TcIF=[1 1 0.25 0.3 0 0 1 1 0.3 0.36 0 0 0 0]  GHd=[66 66 233]  TcHF="[0.01 0.012 0 0 0 0  0.012 0.0144 0 0 0 0 1 1]"  LIM=[.075 .15 .15 .15]  Plot_On=off  MagdB_On=off  FreqRange=logspace(-2,2,500)
  Machine 2 Measurement Demux : powerlib/Machines/Machines Measurement Demux  machType=Synchronous  ssm1=on  ssm2=on  ssm3=on  ssm4=on  ssm5=on  ssm6=on  sm1=off  sm2=off  sm3=off  sm4=off  sm5=off  sm6=on  sm7=on  sm8=on  sm9=on  sm10=on  sm11=on  sm115=off  sm12=off  sm13=off  sm14=off  asm1=on  asm2=on  asm3=on  asm4=on  asm5=on  asm6=on  asm7=on  asm8=on  asm9=on  asm10=on  asm11=on  pmsm1=on  pmsm2=on  pmsm3=on  pmsm4=on  pmsm5=on  pmsm6=on  lastType=2
  Multiport Switch : MultiPortSwitch  InputSameDT=on
  PSS model1 : Constant  Value=0
  PSS model2 : Constant
  Real-Imag to Complex : RealImagToComplex
  STG : powerlib/Machines/Steam Turbine and Governor  gentype=Tandem-compound (single mass)  reg1="[ 1  0.05    0 ]"  reg2="[ 0.001  0.15 ]"  reg3="[ -0.1  0.1  0  4.496 ]"  turb1="[ 0  10   3.3   0.5   ]"  turb2="[   0   0.36    0.36   0.28   ]"  HA="[ 0.046  1.430  1.465   0.192 ]"  KA="[ 90.44  53.88  64.59   62.94  ]"  DA="[ 0.0115  0.3575  0.3663   0.0137  ]"  ini1=0.7777  ini2=[0.779243,-42.8075]
  Sum1 : Sum  SaturateOnIntegerOverflow=on  InputSameDT=on
  Sum2 : Sum  Inputs=-+  SaturateOnIntegerOverflow=on  InputSameDT=on
  Terminator : Terminator
  Terminator1 : Terminator
  Terminator2 : Terminator
  wref : Constant
  Pm : Outport  InitialOutput=0
  Vf : Outport  Port=2  InitialOutput=0
  tag scope: EFD2=global, Pa2=global, Pe2=global, Vt2=global, pss2=global, theta2=global, w2=global
  wires:
  Sum2/1 -> [Pa2], "Delta Pa PSS "/1  "Pm-Pe"
  Machine 2 Measurement Demux/5 -> "MB-PSS "/1, "Delta w PSS (Kundur) "/1
  Machine 2 Measurement Demux/4 -> Sum2/1, [Pe2]
  Machine 2 Measurement Demux/3 -> [w2], STG/3
  Machine 2 Measurement Demux/1 -> Demux/1
  PSS/1 -> Sum1/1
  Sum1/1 -> Multiport Switch/1
  PSS model2/1 -> Sum1/2
  "Delta Pa PSS "/1 -> Multiport Switch/5
  "Delta w PSS (Kundur) "/1 -> Multiport Switch/4
  "MB-PSS "/1 -> Multiport Switch/3
  PSS model1/1 -> Multiport Switch/2
  Multiport Switch/1 -> [pss2], EXCITATION/4
  Machine 2 Measurement Demux/6 -> [theta2]
  Complex to Magnitude-Angle/1 -> [Vt2]
  EXCITATION/1 -> [EFD2], Vf/1
  Real-Imag to Complex/1 -> Complex to Magnitude-Angle/1
  Vref/1 -> EXCITATION/1
  m/1 -> Machine 2 Measurement Demux/1
  Pref/1 -> STG/2
  wref/1 -> STG/1
  Demux/2 -> EXCITATION/3, Real-Imag to Complex/2
  Demux/1 -> EXCITATION/2, Real-Imag to Complex/1
  STG/1 -> Terminator/1
  STG/2 -> Terminator1/1
  STG/3 -> Terminator2/1
  STG/4 -> Pm/1, Sum2/2
  Machine 2 Measurement Demux/2 -> STG/4

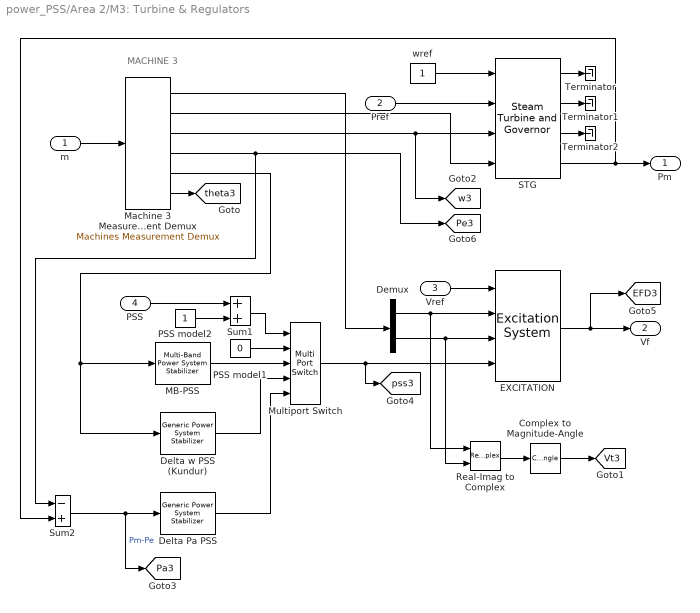
== system power_PSS/Area 2/M3: Turbine & Regulators ==
  note: MACHINE 3
  m : Inport  Port=1  LatchInput=off
  Pref : Inport  Port=2  LatchInput=off
  Vref : Inport  Port=3  LatchInput=off
  PSS : Inport  Port=4  LatchInput=off
  Complex to Magnitude-Angle : ComplexToMagnitudeAngle  Output=Magnitude
  "Delta Pa PSS " : powerlib/Machines/Generic Power System Stabilizer  Tsensor=15e-3  K=2.5*1.25  Twashout=1  Tleadlag1=[60e-3 1]  Tleadlag2=[0 0]  VSlimits=[-0.15 0.15]  Vinit=0  Plot_On=off  MagdB_On=on  FreqRange=logspace(-2,2,500)
  "Delta w PSS (Kundur) " : powerlib/Machines/Generic Power System Stabilizer  Tsensor=15e-3  K=30  Twashout=10  Tleadlag1=[50e-3 20e-3]  Tleadlag2=[3 5.4]  VSlimits=[-0.15 0.15]  Vinit=0  Plot_On=off  MagdB_On=on  FreqRange=logspace(-2,2,500)
  Demux : Demux  Outputs=2
  EXCITATION : powerlib/Machines/Excitation System  tr=20e-3  reg=[ 200, 0.001 ]  exc=[ 1, 0 ]  tgr=[ 0, 0 ]  damp=[ 0, 0 ]  sat=[ 0, 0 ]  lim=[ 0 , 12.3, 0 ]  v0=[1,1.85092]
  "MB-PSS " : powerlib/Machines/Multi-Band Power System Stabilizer  OperationMode=Simplified settings  Kg=1.0  GL=[0.2 30]  GI=[1.25 40]  GH=[12.0 160]  GLd=[66 66 9.4]  TcLF=[1.667 2 0 0 0 0 2 2.4 0 0 0 0 1 1]  GId=[66 66 47.6]  TcIF=[1 1 0.25 0.3 0 0 1 1 0.3 0.36 0 0 0 0]  GHd=[66 66 233]  TcHF="[0.01 0.012 0 0 0 0  0.012 0.0144 0 0 0 0 1 1]"  LIM=[.075 .15 .15 .15]  Plot_On=off  MagdB_On=off  FreqRange=logspace(-2,2,500)
  Machine 3 Measurement Demux : powerlib/Machines/Machines Measurement Demux  machType=Synchronous  ssm1=on  ssm2=on  ssm3=on  ssm4=on  ssm5=on  ssm6=on  sm1=off  sm2=off  sm3=off  sm4=off  sm5=off  sm6=on  sm7=on  sm8=on  sm9=on  sm10=on  sm11=on  sm115=off  sm12=off  sm13=off  sm14=off  asm1=on  asm2=on  asm3=on  asm4=on  asm5=on  asm6=on  asm7=on  asm8=on  asm9=on  asm10=on  asm11=on  pmsm1=on  pmsm2=on  pmsm3=on  pmsm4=on  pmsm5=on  pmsm6=on  lastType=2
  Multiport Switch : MultiPortSwitch  InputSameDT=on
  PSS model1 : Constant  Value=0
  PSS model2 : Constant
  Real-Imag to Complex : RealImagToComplex
  STG : powerlib/Machines/Steam Turbine and Governor  gentype=Tandem-compound (single mass)  reg1="[ 1  0.05    0 ]"  reg2="[ 0.001  0.15 ]"  reg3="[ -0.1  0.1  0  4.496 ]"  turb1="[ 0  10   3.3   0.5   ]"  turb2="[   0   0.36    0.36   0.28   ]"  HA="[ 0.046  1.430  1.465   0.192 ]"  KA="[ 90.44  53.88  64.59   62.94  ]"  DA="[ 0.0115  0.3575  0.3663   0.0137  ]"  ini1=0.798889  ini2=[0.800505,-56.3243]
  Sum1 : Sum  SaturateOnIntegerOverflow=on  InputSameDT=on
  Sum2 : Sum  Inputs=-+  SaturateOnIntegerOverflow=on  InputSameDT=on
  Terminator : Terminator
  Terminator1 : Terminator
  Terminator2 : Terminator
  wref : Constant
  Pm : Outport  InitialOutput=0
  Vf : Outport  Port=2  InitialOutput=0
  tag scope: EFD3=global, Pa3=global, Pe3=global, Vt3=global, pss3=global, theta3=global, w3=global
  wires:
  Sum2/1 -> [Pa3], "Delta Pa PSS "/1  "Pm-Pe"
  Machine 3 Measurement Demux/5 -> "MB-PSS "/1, "Delta w PSS (Kundur) "/1
  Machine 3 Measurement Demux/4 -> Sum2/1, [Pe3]
  Machine 3 Measurement Demux/3 -> [w3], STG/3
  Machine 3 Measurement Demux/1 -> Demux/1
  PSS/1 -> Sum1/1
  Sum1/1 -> Multiport Switch/1
  PSS model2/1 -> Sum1/2
  "Delta Pa PSS "/1 -> Multiport Switch/5
  "Delta w PSS (Kundur) "/1 -> Multiport Switch/4
  "MB-PSS "/1 -> Multiport Switch/3
  PSS model1/1 -> Multiport Switch/2
  Multiport Switch/1 -> [pss3], EXCITATION/4
  Machine 3 Measurement Demux/6 -> [theta3]
  Complex to Magnitude-Angle/1 -> [Vt3]
  EXCITATION/1 -> [EFD3], Vf/1
  Real-Imag to Complex/1 -> Complex to Magnitude-Angle/1
  Vref/1 -> EXCITATION/1
  m/1 -> Machine 3 Measurement Demux/1
  Pref/1 -> STG/2
  wref/1 -> STG/1
  Demux/2 -> EXCITATION/3, Real-Imag to Complex/2
  Demux/1 -> EXCITATION/2, Real-Imag to Complex/1
  Machine 3 Measurement Demux/2 -> STG/4
  STG/1 -> Terminator/1
  STG/2 -> Terminator1/1
  STG/3 -> Terminator2/1
  STG/4 -> Pm/1, Sum2/2

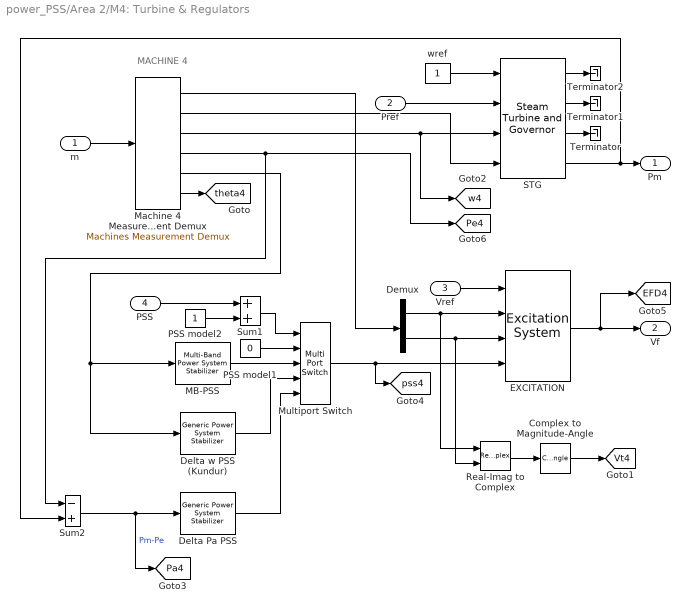
== system power_PSS/Area 2/M4: Turbine & Regulators ==
  note: MACHINE 4
  m : Inport  Port=1  LatchInput=off
  Pref : Inport  Port=2  LatchInput=off
  Vref : Inport  Port=3  LatchInput=off
  PSS : Inport  Port=4  LatchInput=off
  Complex to Magnitude-Angle : ComplexToMagnitudeAngle  Output=Magnitude
  "Delta Pa PSS " : powerlib/Machines/Generic Power System Stabilizer  Tsensor=15e-3  K=2.5*1.25  Twashout=1  Tleadlag1=[60e-3 1]  Tleadlag2=[0 0]  VSlimits=[-0.15 0.15]  Vinit=0  Plot_On=off  MagdB_On=on  FreqRange=logspace(-2,2,500)
  "Delta w PSS (Kundur) " : powerlib/Machines/Generic Power System Stabilizer  Tsensor=15e-3  K=30  Twashout=10  Tleadlag1=[50e-3 20e-3]  Tleadlag2=[3 5.4]  VSlimits=[-0.15 0.15]  Vinit=0  Plot_On=off  MagdB_On=on  FreqRange=logspace(-2,2,500)
  Demux : Demux  Outputs=2
  EXCITATION : powerlib/Machines/Excitation System  tr=20e-3  reg=[ 200, 0.001 ]  exc=[ 1, 0 ]  tgr=[ 0, 0 ]  damp=[ 0, 0 ]  sat=[ 0, 0 ]  lim=[ 0 , 12.3, 0 ]  v0=[1,1.82209]
  "MB-PSS " : powerlib/Machines/Multi-Band Power System Stabilizer  OperationMode=Simplified settings  Kg=1.0  GL=[0.2 30]  GI=[1.25 40]  GH=[12.0 160]  GLd=[66 66 9.4]  TcLF=[1.667 2 0 0 0 0 2 2.4 0 0 0 0 1 1]  GId=[66 66 47.6]  TcIF=[1 1 0.25 0.3 0 0 1 1 0.3 0.36 0 0 0 0]  GHd=[66 66 233]  TcHF="[0.01 0.012 0 0 0 0  0.012 0.0144 0 0 0 0 1 1]"  LIM=[.075 .15 .15 .15]  Plot_On=off  MagdB_On=off  FreqRange=logspace(-2,2,500)
  Machine 4 Measurement Demux : powerlib/Machines/Machines Measurement Demux  machType=Synchronous  ssm1=on  ssm2=on  ssm3=on  ssm4=on  ssm5=on  ssm6=on  sm1=off  sm2=off  sm3=off  sm4=off  sm5=off  sm6=on  sm7=on  sm8=on  sm9=on  sm10=on  sm11=on  sm115=off  sm12=off  sm13=off  sm14=off  asm1=on  asm2=on  asm3=on  asm4=on  asm5=on  asm6=on  asm7=on  asm8=on  asm9=on  asm10=on  asm11=on  pmsm1=on  pmsm2=on  pmsm3=on  pmsm4=on  pmsm5=on  pmsm6=on  lastType=2
  Multiport Switch : MultiPortSwitch  InputSameDT=on
  PSS model1 : Constant  Value=0
  PSS model2 : Constant
  Real-Imag to Complex : RealImagToComplex
  STG : powerlib/Machines/Steam Turbine and Governor  gentype=Tandem-compound (single mass)  reg1="[ 1  0.05    0 ]"  reg2="[ 0.001  0.15 ]"  reg3="[ -0.1  0.1  0  4.496 ]"  turb1="[ 0  10   3.3   0.5   ]"  turb2="[   0   0.36    0.36   0.28   ]"  HA="[ 0.046  1.430  1.465   0.192 ]"  KA="[ 90.44  53.88  64.59   62.94  ]"  DA="[ 0.0115  0.3575  0.3663   0.0137  ]"  ini1=0.7778  ini2=[0.779311,-67.7513]
  Sum1 : Sum  SaturateOnIntegerOverflow=on  InputSameDT=on
  Sum2 : Sum  Inputs=-+  SaturateOnIntegerOverflow=on  InputSameDT=on
  Terminator : Terminator
  Terminator1 : Terminator
  Terminator2 : Terminator
  wref : Constant
  Pm : Outport  InitialOutput=0
  Vf : Outport  Port=2  InitialOutput=0
  tag scope: EFD4=global, Pa4=global, Pe4=global, Vt4=global, pss4=global, theta4=global, w4=global
  wires:
  Demux/1 -> Real-Imag to Complex/1, EXCITATION/2
  Demux/2 -> Real-Imag to Complex/2, EXCITATION/3
  STG/4 -> Pm/1, Sum2/2
  wref/1 -> STG/1
  Pref/1 -> STG/2
  m/1 -> Machine 4 Measurement Demux/1
  Vref/1 -> EXCITATION/1
  STG/3 -> Terminator/1
  Real-Imag to Complex/1 -> Complex to Magnitude-Angle/1
  EXCITATION/1 -> Vf/1, [EFD4]
  Complex to Magnitude-Angle/1 -> [Vt4]
  Machine 4 Measurement Demux/6 -> [theta4]
  Multiport Switch/1 -> EXCITATION/4, [pss4]
  PSS model1/1 -> Multiport Switch/2
  "MB-PSS "/1 -> Multiport Switch/3
  "Delta w PSS (Kundur) "/1 -> Multiport Switch/4
  "Delta Pa PSS "/1 -> Multiport Switch/5
  PSS model2/1 -> Sum1/2
  Sum1/1 -> Multiport Switch/1
  PSS/1 -> Sum1/1
  Machine 4 Measurement Demux/1 -> Demux/1
  Machine 4 Measurement Demux/3 -> [w4], STG/3
  Machine 4 Measurement Demux/4 -> Sum2/1, [Pe4]
  Machine 4 Measurement Demux/5 -> "MB-PSS "/1, "Delta w PSS (Kundur) "/1
  Sum2/1 -> [Pa4], "Delta Pa PSS "/1  "Pm-Pe"
  STG/2 -> Terminator1/1
  STG/1 -> Terminator2/1
  Machine 4 Measurement Demux/2 -> STG/4
